simulink library "controlLibrary"  (R2023a)
settings: Solver=VariableStepAuto  StartTime=0.0  StopTime=10.0  RelTol=1e-3
undefined symbols (not defined in the file): Up
libraries: dspswit3 x1, simulink x1
settings Model: Creator=mwalker  LastModifiedBy=ppatel
settings SolverCC: AlgebraicLoopSolver=TrustRegion
settings DebuggingCC: UnconnectedInputMsg=warning  UnconnectedOutputMsg=warning  UnconnectedLineMsg=warning
settings ModelReferenceCC: EnableRefExpFcnMdlSchedulingChecks=on

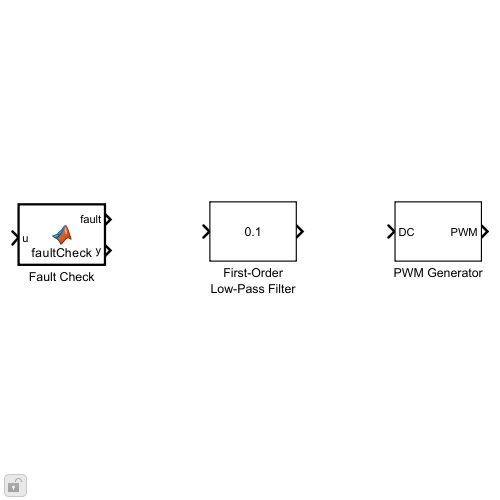
[thumbnail: Simulink's stored preview of the top-level diagram]
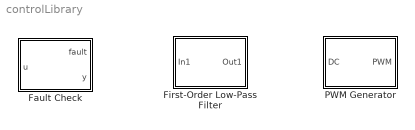
== system controlLibrary ==
  Fault Check : MATLAB Function  TreatAsAtomicUnit=on
  First-Order Low-Pass Filter : Subsystem  mask(First-Order Low-Pass Filter){fc=0.1}
      mask prompts: fc "Filter Constant"
      mask Display: disp(get_param(gcb,'fc'))
  PWM Generator : Subsystem  mask(PWM Generator){CarrCount=Up, Tper=0.001/0.05, Ts=0.001}
      mask prompts: CarrCount "Carrier counter:"; Tper "Timer period (s):"; Ts "Sample time"
      mask help:
      | This block implements a PWM generator.
      |
      | For discrete-time, set Sample time to a positive value. For continuous-time, set Sample time to zero.
      mask TypeOptions CarrCount: Carrier counter/CarrCount
      mask TypeOptions Tper: Carrier counter/Tper
      mask TypeOptions Ts: Carrier counter/Ts

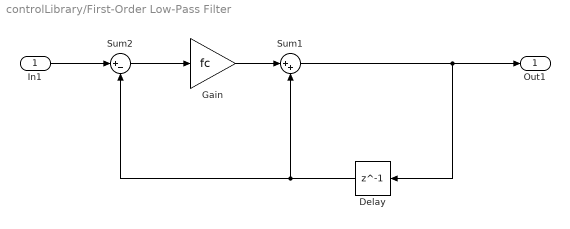
== system controlLibrary/First-Order Low-Pass Filter ==
  In1 : Inport
  Delay : Delay  DelayLength=1  InitialCondition=0
  Gain : Gain  Gain=fc
  Sum1 : Sum  Inputs=|++
  Sum2 : Sum  Inputs=|+-
  Out1 : Outport
  wires:
  In1/1 -> Sum2/1
  Sum1/1 -> Out1/1, Delay/1
  Sum2/1 -> Gain/1
  Delay/1 -> Sum2/2, Sum1/2
  Gain/1 -> Sum1/1

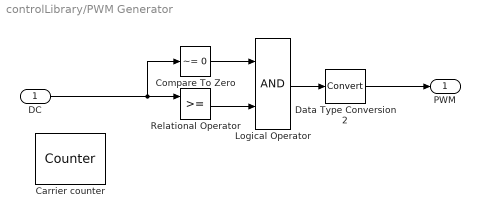
== system controlLibrary/PWM Generator ==
  DC : Inport  SampleTime=Ts
  Carrier counter : dspswit3/Counter  Direction=Up  CountEvent=Rising edge  CounterSize=User defined  MaxCount=255  InitialCount=0  Output=Count and Hit  HitValue=32  ResetInput=on  SamplesPerFrame=1  Ts=Ts  CntDtype=double  HitDtype=Logical
  Compare To Zero : simulink/Logic and Bit Operations/Compare To Zero  relop=~=  OutDataTypeStr=boolean
  Data Type Conversion2 : DataTypeConversion  SaturateOnIntegerOverflow=off  RndMeth=Floor
  Logical Operator : Logic  AllPortsSameDT=off  OutDataTypeStr=boolean
  Relational Operator : RelationalOperator  OutDataTypeStr=boolean  RndMeth=Simplest  InputSameDT=off
  PWM : Outport  VectorParamsAs1DForOutWhenUnconnected=off
  wires:
  ? -> Relational Operator/2
  Logical Operator/1 -> Data Type Conversion2/1
  Compare To Zero/1 -> Logical Operator/1
  Relational Operator/1 -> Logical Operator/2
  DC/1 -> Compare To Zero/1, Relational Operator/1
  Data Type Conversion2/1 -> PWM/1

== matlab function controlLibrary/Fault Check ==
  data: u input; fault output; y output
function [fault,y] = faultCheck(u)

if u > single(4.5) || u < single(0.5)
    fault = true;
    y = single(2.5); % Choose an appropriate default value
else
    fault = false;
    y = u; % Pass the input through
end
